simulink model "Final_Implementation"  (R2025b)
settings: Solver=ode4  StartTime=0.0  StopTime=10.0  FixedStep=2e-4  RelTol=1e-3  EnableMultiTasking=on
undefined symbols (not defined in the file or in its folder): P, Q_local, Q_opt_scaled, Q_OPT_scaled, T_S, x_0
libraries: simulink x4, dspsigops x3, SignalEditorBlockLib x1
settings Model: SimulationMode=rapid-accelerator  SILPILSystemUnderTest=refmodels  SILPILSimulationModeTopModel=rapid-accelerator  CodeVerificationMode=processor-in-the-loop (pil)  ExtModeTrigDuration=2  ExplicitPartitioning=on  Creator=nabil  LastModifiedBy=ouka1
settings SolverCC: AllowMultiTaskInputOutput=on  ConcurrentTasks=on  PositivePriorityOrder=on  AutoInsertRateTranBlk=on
settings OptimizationCC: StrengthReduction=on  PassReuseOutputArgsAs=Individual arguments  ZeroExternalMemoryAtStartup=off  ZeroInternalMemoryAtStartup=off  MaxStackSize=200000  OptimizeBlockOrder=speed  OptimizationPriority=Speed  OptimizationCustomize=off  MultiThreadedLoops=on  AutoScheduleForLoops=on  EfficientTunableParamExpr=on
settings DebuggingCC: ParameterTunabilityLossMsg=error
settings HardwareCC: ProdBitPerLong=64.0  ProdLargestAtomicInteger=LongLong  ProdLargestAtomicFloat=Double  ProdLongLongMode=on  ProdHWDeviceType=ARM Compatible->ARM Cortex-A (64-bit)
settings ModelReferenceCC: PropagateVarSize=During execution
settings SFSimCC: SimUserIncludeDirs=./Simulation_ert_rtw/
settings SFSimCC: SimUserSources=|
  | functions.c
  | Simulation.c
  | Simulation_data.c
settings RTWCC: SystemTargetFile=ert.tlc  HardwareBoard=Raspberry Pi (64bit)  TLCOptions="-aInlineSetEventsForThisBaseRateFcn=TLC_FALSE -aSuppressMultiTaskScheduler=TLC_FALSE  -aRateBasedStepFcn=0"  TemplateMakefile=ert_default_tmf  CustomInclude=./Simulation_ert_rtw/  Toolchain=GNU GCC Embedded Linux  BuildConfiguration=Faster Runs  IncludeHyperlinkInReport=on  GenerateCodeMetricsReport=on  Description=Embedded Coder
settings RTWCC: CustomHeaderCode=|
  | functions.h
  | Simulation.h
settings RTWCC: CustomSource=|
  | functions.c
  | Simulation.c
settings CodeAppCC: ForceParamTrailComments=on  IgnoreCustomStorageClasses=off  OperatorAnnotations=on  SimulinkDataObjDesc=on  SFDataObjDesc=on  InsertBlockDesc=on
settings ERTTargetCC: ExtModeTransport=2.0  ExtModeStaticAlloc=on  ExtModeMexFile=ext_xcp  ExtModeIntrfLevel=Level2 - Open  InlinedParameterPlacement=Hierarchical  CodeReplacementLibrary=ARM Cortex-A CMSIS  SupportNonFinite=off  SupportVariableSizeSignals=on  InstructionSetFMA=on  OptimizeReductions=on

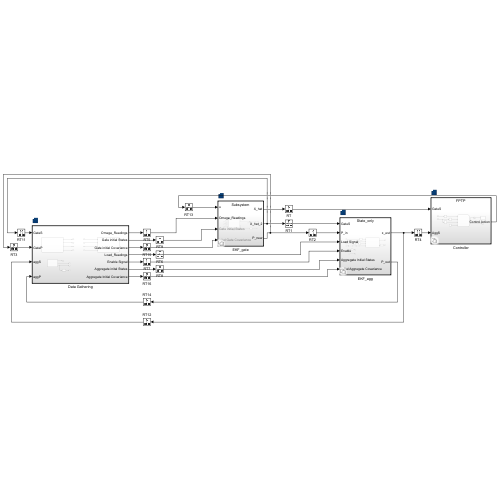
[thumbnail: Simulink's stored preview of the top-level diagram]
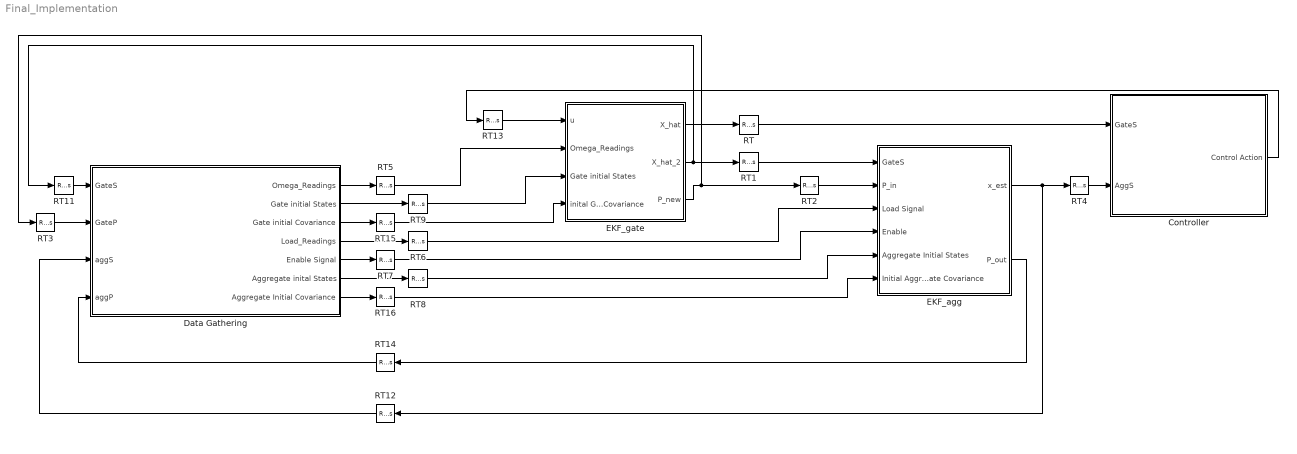
== system Final_Implementation ==
  Controller : Subsystem  TreatAsAtomicUnit=on  Variant=on  EmptyChoice=on
  Data Gathering : Subsystem  TreatAsAtomicUnit=on  SystemSampleTime=2e-3
  EKF_agg : Subsystem  TreatAsAtomicUnit=on  Variant=on  EmptyChoice=on
  EKF_gate : Subsystem  TreatAsAtomicUnit=on  Variant=on  EmptyChoice=on
  RT : RateTransition  Deterministic=off  OutPortSampleTime=0.005
  RT{1..2,6..8,16} (6 alike) : RateTransition  Deterministic=off  OutPortSampleTime=0.001
  RT{3,11..12,14} (4 alike) : RateTransition  Deterministic=off  OutPortSampleTime=0.002
  RT{5,9,13,15} (4 alike) : RateTransition  Deterministic=off  OutPortSampleTime=0.0002
  RT4 : RateTransition  Deterministic=off  OutPortSampleTime=0.005
  wires:
  Data Gathering/1(Omega_Readings) -> RT5/1
  Data Gathering/4(Load_Readings) -> RT6/1
  Data Gathering/5(Enable Signal) -> RT7/1
  Data Gathering/6(Aggregate inital States) -> RT8/1
  Data Gathering/2(Gate initial States) -> RT9/1
  RT11/1 -> Data Gathering/1(GateS)
  RT12/1 -> Data Gathering/3(aggS)
  RT3/1 -> Data Gathering/2(GateP)
  RT14/1 -> Data Gathering/4(aggP)
  Data Gathering/3(Gate initial Covariance) -> RT15/1
  Data Gathering/7(Aggregate Initial Covariance) -> RT16/1
  RT/1 -> Controller/1(GateS)
  RT4/1 -> Controller/2(AggS)
  Controller/1(Control Action) -> RT13/1
  RT1/1 -> EKF_agg/1(GateS)
  RT2/1 -> EKF_agg/2(P_in)
  RT6/1 -> EKF_agg/3(Load Signal)
  RT7/1 -> EKF_agg/4(Enable)
  RT8/1 -> EKF_agg/5(Aggregate Initial States)
  RT16/1 -> EKF_agg/6(Initial Aggregate Covariance)
  EKF_agg/1(x_est) -> RT4/1, RT12/1
  EKF_agg/2(P_out) -> RT14/1
  RT13/1 -> EKF_gate/1(u)
  RT5/1 -> EKF_gate/2(Omega_Readings)
  RT9/1 -> EKF_gate/3(Gate initial States)
  RT15/1 -> EKF_gate/4(inital Gate Covariance)
  EKF_gate/1(X_hat) -> RT/1
  EKF_gate/2(X_hat_2) -> RT1/1, RT11/1
  EKF_gate/3(P_new) -> RT2/1, RT3/1

== system Final_Implementation/Controller ==
  GateS : Inport
  AggS : Inport  Port=2
  FPTP : Subsystem  VariantControl=Controller==1
  MPC : Subsystem  TreatAsAtomicUnit=on  SystemSampleTime=0.005  VariantControl=Controller==0
  Control Action : Outport

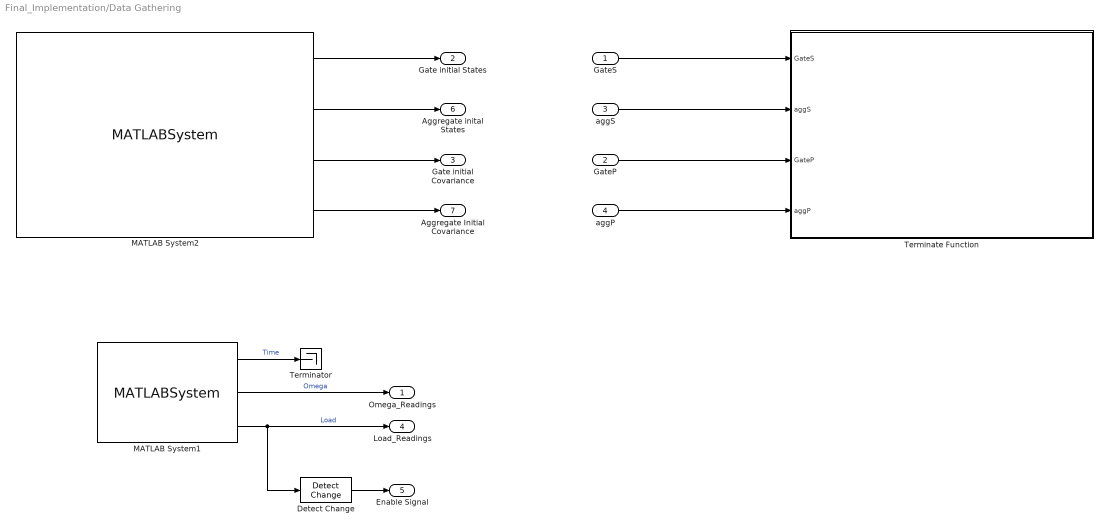
== system Final_Implementation/Data Gathering ==
  GateS : Inport
  GateP : Inport  Port=2
  aggS : Inport  Port=3
  aggP : Inport  Port=4
  Detect Change : simulink/Logic and Bit Operations/Detect Change  vinit=0  OutDataTypeStr=boolean
  MATLAB System1 : MATLABSystem  System=SerialReadBlock  SimulateUsing=Code generation
      mask Type: SerialReadBlock
  MATLAB System2 : MATLABSystem  System=LastStateInitializer  FileName=sim_data.csv  SimulateUsing=Code generation
      mask Type: LastStateInitializer
  Terminate Function : Subsystem  TreatAsAtomicUnit=on
  Terminator : Terminator
  Omega_Readings : Outport
  Gate initial States : Outport  Port=2
  Gate initial Covariance : Outport  Port=3
  Load_Readings : Outport  Port=4
  Enable Signal : Outport  Port=5
  Aggregate inital States : Outport  Port=6
  Aggregate Initial Covariance : Outport  Port=7
  wires:
  MATLAB System1/2 -> Omega_Readings/1  "Omega"
  MATLAB System1/3 -> Detect Change/1, Load_Readings/1  "Load"
  Detect Change/1 -> Enable Signal/1
  MATLAB System2/1 -> Gate initial States/1
  MATLAB System2/2 -> Aggregate inital States/1
  MATLAB System2/3 -> Gate initial Covariance/1
  MATLAB System2/4 -> Aggregate Initial Covariance/1
  aggS/1 -> Terminate Function/2(aggS)
  GateP/1 -> Terminate Function/3(GateP)
  GateS/1 -> Terminate Function/1(GateS)
  aggP/1 -> Terminate Function/4(aggP)
  MATLAB System1/1 -> Terminator/1  "Time"

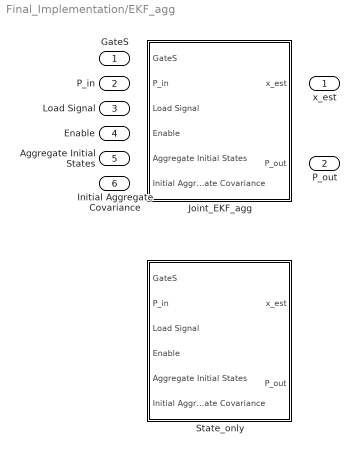
== system Final_Implementation/EKF_agg ==
  GateS : Inport
  P_in : Inport  Port=2
  Load Signal : Inport  Port=3
  Enable : Inport  Port=4
  Aggregate Initial States : Inport  Port=5
  Initial Aggregate Covariance : Inport  Port=6
  Joint_EKF_agg : Subsystem  TreatAsAtomicUnit=on  SystemSampleTime=1e-3  VariantControl=Estimator==0
  State_only : Subsystem  TreatAsAtomicUnit=on  VariantControl=Estimator==1
  x_est : Outport
  P_out : Outport  Port=2

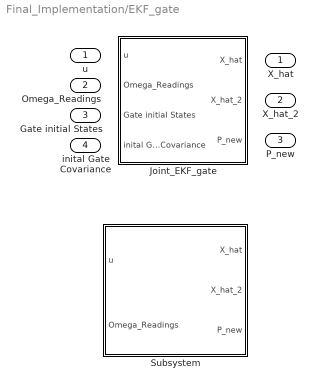
== system Final_Implementation/EKF_gate ==
  u : Inport
  Omega_Readings : Inport  Port=2
  Gate initial States : Inport  Port=3
  inital Gate Covariance : Inport  Port=4
  Joint_EKF_gate : Subsystem  TreatAsAtomicUnit=on  SystemSampleTime=2e-4  VariantControl=Estimator==0
  Subsystem : Subsystem  TreatAsAtomicUnit=on  VariantControl=Estimator==1
  X_hat : Outport
  X_hat_2 : Outport  Port=2
  P_new : Outport  Port=3

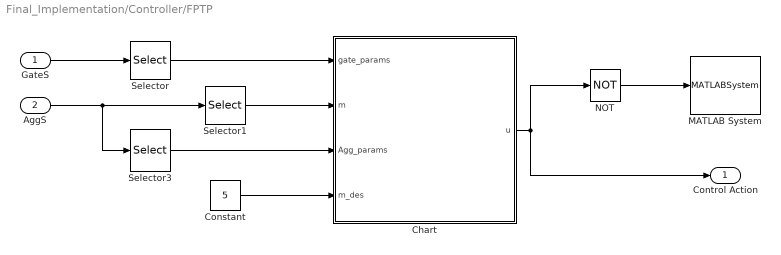
== system Final_Implementation/Controller/FPTP ==
  GateS : Inport
  AggS : Inport  Port=2
  Chart : Stateflow chart  TreatAsAtomicUnit=on
      settings: PortSchema="{\"entries\":[{\"content\":{\"sides\":[{\"content\":{\"connectorIds\":[\"In1\",\"In3\",\"In2\",\"In4\"]},\"type\":\"ConnectorPlacement.EquallySpacedRectSide\",\"uuid\":\"c09b967c-3e4e-4bac-bda4-fda1bd96a736\"},{\"content\":{\"connectorIds\":[\"Out1\"],\"side\":\"RIGHT\"},\"type\":\"ConnectorPlacement.EquallySpacedRectSide\",\"uuid\":\"db87db1d-7eac-4fd3-9563-2d6b00b990a6\"},{\"content\":{\"side\":\"TOP\"},\"type\":\"ConnectorPlacement.EquallySpacedRectSide\",\"uuid\":\"64da0432-1b95-42e2-a853-d892c1769434\"}]},\"type\":\"ConnectorPlacement.EquallySpacedConnector\",\"uuid\":\"e785f849-6cb9-45a7-bfa8-d41e67ce6963\"}],\"packageUris\":[\"http://schema.mathworks.com/mf0/Connector/R2020b\"],\"version\":\"1.0\"}"
  Constant : Constant  Value=5
  MATLAB System : MATLABSystem  System=GateDriver  SimulateUsing=Code generation
      mask Type: GateDriver
  NOT : Logic  Operator=NOT  IconShape=distinctive  AllPortsSameDT=off  OutDataTypeStr=boolean
  Selector : Selector  InputPortWidth=6  IndexOptions=Index vector (dialog)  Indices=[5 6]  OutputSizes=1
  Selector1 : Selector  InputPortWidth=9  IndexOptions=Index vector (dialog)  Indices=2  OutputSizes=1
  Selector3 : Selector  InputPortWidth=9  IndexOptions=Index vector (dialog)  Indices=[5:9]  OutputSizes=1
  Control Action : Outport
  wires:
  GateS/1 -> Selector/1
  Selector/1 -> Chart/1(gate_params)
  AggS/1 -> Selector3/1, Selector1/1
  Selector1/1 -> Chart/3(m)
  Constant/1 -> Chart/4(m_des)
  Selector3/1 -> Chart/2(Agg_params)
  NOT/1 -> MATLAB System/1
  Chart/1(u) -> NOT/1, Control Action/1

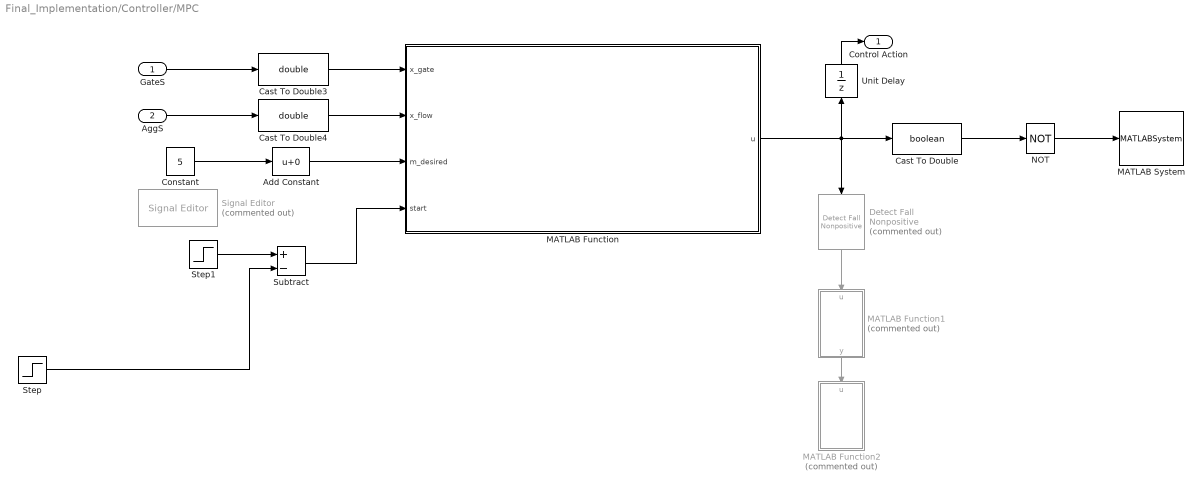
== system Final_Implementation/Controller/MPC ==
  GateS : Inport
  AggS : Inport  Port=2
  Add Constant : Bias  SaturateOnIntegerOverflow=off
  Cast To Double : DataTypeConversion  OutDataTypeStr=boolean  SaturateOnIntegerOverflow=off  RndMeth=Floor
  Cast To Double3 : DataTypeConversion  OutDataTypeStr=double  SaturateOnIntegerOverflow=off  RndMeth=Floor
  Cast To Double4 : DataTypeConversion  OutDataTypeStr=double  SaturateOnIntegerOverflow=off  RndMeth=Floor
  Constant : Constant  Value=5
  Detect Fall Nonpositive : simulink/Logic and Bit Operations/Detect Fall Nonpositive  Commented=on  vinit=0  OutDataTypeStr=boolean
  MATLAB Function : MATLAB Function  TreatAsAtomicUnit=on
  MATLAB Function1 : MATLAB Function  Commented=on  TreatAsAtomicUnit=on
  MATLAB Function2 : MATLAB Function  Commented=on  TreatAsAtomicUnit=on
  MATLAB System : MATLABSystem  System=GateDriver  SimulateUsing=Code generation
      mask Type: GateDriver
  NOT : Logic  Operator=NOT  IconShape=distinctive  AllPortsSameDT=off  OutDataTypeStr=boolean
  Signal Editor : SignalEditorBlockLib/Signal Editor  Commented=on  FileName=untitled.mat  ActiveScenario=Scenario  ActiveSignal=Signal 1  IsBus=off  OutputBusObjectStr=Bus: BusObject  SampleTime=0.005  ZeroCross=off  OutputAfterFinalValue=Setting to zero  Unit=inherit  PreserveSignalName=on  ApplySigPropsToAllScenarios=on  ApplySigPropsToAllSignals=off  SignalPropertySource=Dialog parameters
  Step : Step  Time=5e-3  Before=1  After=0
  Step1 : Step  Time=15e-3  Before=1  After=0
  Subtract : Sum  Inputs=+-
  Unit Delay : UnitDelay  SampleTime=0.005  HasFrameUpgradeWarning=on
  Control Action : Outport
  wires:
  Cast To Double4/1 -> MATLAB Function/2(x_flow)
  Constant/1 -> Add Constant/1
  Cast To Double3/1 -> MATLAB Function/1(x_gate)
  Unit Delay/1 -> Control Action/1
  AggS/1 -> Cast To Double4/1
  GateS/1 -> Cast To Double3/1
  Cast To Double/1 -> NOT/1
  NOT/1 -> MATLAB System/1
  MATLAB Function/1(u) -> Detect Fall Nonpositive/1, Cast To Double/1, Unit Delay/1
  Detect Fall Nonpositive/1 -> MATLAB Function1/1(u)
  MATLAB Function1/1(y) -> MATLAB Function2/1(u)
  Step1/1 -> Subtract/1
  Step/1 -> Subtract/2
  Subtract/1 -> MATLAB Function/4(start)
  Add Constant/1 -> MATLAB Function/3(m_desired)

== system Final_Implementation/Data Gathering/Terminate Function ==
  GateS : Inport
  aggS : Inport  Port=2
  GateP : Inport  Port=3
  aggP : Inport  Port=4
  Event Listener : EventListener  DisableCoverage=on  EventType=Terminate  EventName=reset
  MATLAB System : MATLABSystem  System=LoggerBlock  SimulateUsing=Code generation
      mask Type: LoggerBlock
  wires:
  GateP/1 -> MATLAB System/3
  aggP/1 -> MATLAB System/4
  GateS/1 -> MATLAB System/1
  aggS/1 -> MATLAB System/2

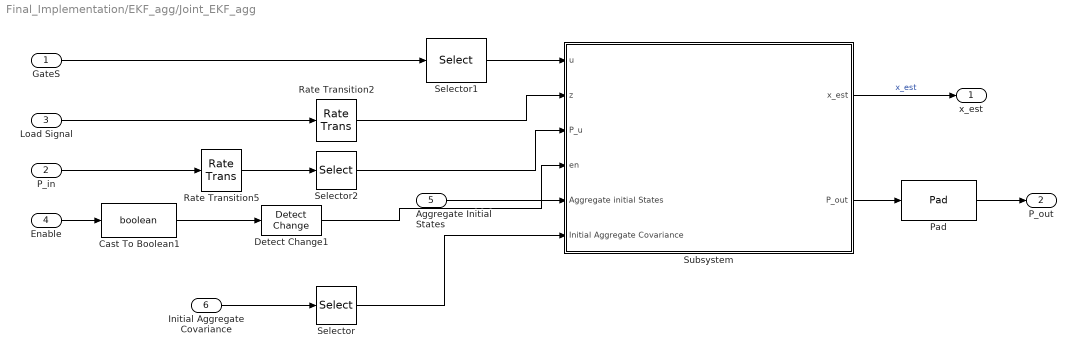
== system Final_Implementation/EKF_agg/Joint_EKF_agg ==
  GateS : Inport
  P_in : Inport  Port=2
  Load Signal : Inport  Port=3
  Enable : Inport  Port=4
  Aggregate Initial States : Inport  Port=5
  Initial Aggregate Covariance : Inport  Port=6
  Cast To Boolean1 : DataTypeConversion  OutDataTypeStr=boolean  SaturateOnIntegerOverflow=off  RndMeth=Floor
  Detect Change1 : simulink/Logic and Bit Operations/Detect Change  vinit=0  OutDataTypeStr=boolean
  Pad : dspsigops/Pad  padAlong=Columns and rows  dimsToPad=1  valSrc=Specify via dialog  padVal=0  spec=Output size  padNumOutRowsSpecMethod=User-specified  numOutRows=9  padNumOutColsSpecMethod=User-specified  numOutCols=9  isVarDimsMode=off  padBeginning=0  padEnd=0  outSizeMode=User-specified  outSize=1  padSigAt=End  trunc_flag=None  roundingMode=Floor  overflowMode=off  truncOrWrapMode=Truncate  wrap_flag=None
  Rate Transition2 : RateTransition
  Rate Transition5 : RateTransition
  Selector : Selector  NumberOfDimensions=2  InputPortWidth=3  IndexOptions=Index vector (dialog),Index vector (dialog)  Indices=[1:7],[1:7]  OutputSizes=1,1
  Selector1 : Selector  InputPortWidth=6  IndexOptions=Index vector (dialog)  Indices=1  OutputSizes=1
  Selector2 : Selector  NumberOfDimensions=2  InputPortWidth=7,7  IndexOptions=Index vector (dialog),Index vector (dialog)  Indices=1,1  OutputSizes=1,1
  Subsystem : Subsystem
  x_est : Outport
  P_out : Outport  Port=2
  wires:
  Subsystem/1(x_est) -> x_est/1  "x_est"
  Subsystem/2(P_out) -> Pad/1
  Enable/1 -> Cast To Boolean1/1
  Rate Transition2/1 -> Subsystem/2(z)
  Cast To Boolean1/1 -> Detect Change1/1
  P_in/1 -> Rate Transition5/1
  Rate Transition5/1 -> Selector2/1
  Selector1/1 -> Subsystem/1(u)
  Load Signal/1 -> Rate Transition2/1
  Detect Change1/1 -> Subsystem/4(en)
  Selector2/1 -> Subsystem/3(P_u)
  Aggregate Initial States/1 -> Subsystem/5(Aggregate initial States)
  GateS/1 -> Selector1/1
  Initial Aggregate Covariance/1 -> Selector/1
  Selector/1 -> Subsystem/6(Initial Aggregate Covariance)
  Pad/1 -> P_out/1

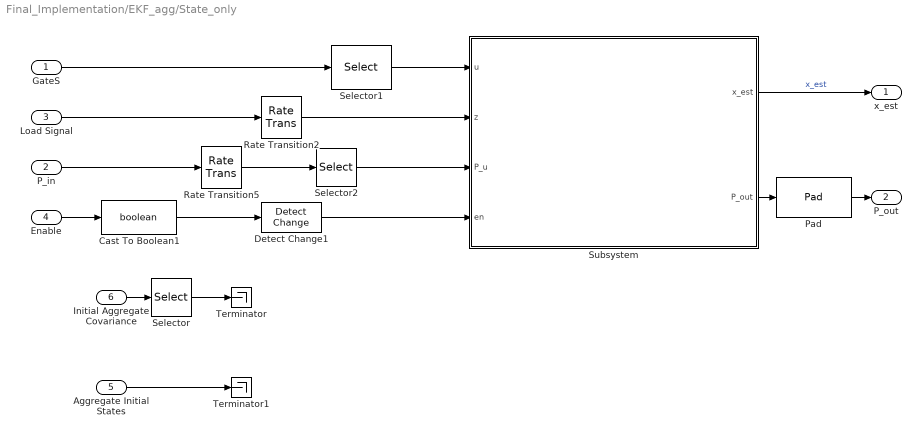
== system Final_Implementation/EKF_agg/State_only ==
  GateS : Inport
  P_in : Inport  Port=2
  Load Signal : Inport  Port=3
  Enable : Inport  Port=4
  Aggregate Initial States : Inport  Port=5
  Initial Aggregate Covariance : Inport  Port=6
  Cast To Boolean1 : DataTypeConversion  OutDataTypeStr=boolean  SaturateOnIntegerOverflow=off  RndMeth=Floor
  Detect Change1 : simulink/Logic and Bit Operations/Detect Change  vinit=0  OutDataTypeStr=boolean
  Pad : dspsigops/Pad  padAlong=Columns and rows  dimsToPad=1  valSrc=Specify via dialog  padVal=0  spec=Output size  padNumOutRowsSpecMethod=User-specified  numOutRows=9  padNumOutColsSpecMethod=User-specified  numOutCols=9  isVarDimsMode=off  padBeginning=0  padEnd=0  outSizeMode=User-specified  outSize=1  padSigAt=End  trunc_flag=None  roundingMode=Floor  overflowMode=off  truncOrWrapMode=Truncate  wrap_flag=None
  Rate Transition2 : RateTransition
  Rate Transition5 : RateTransition
  Selector : Selector  NumberOfDimensions=2  InputPortWidth=3  IndexOptions=Index vector (dialog),Index vector (dialog)  Indices=[1:4],[1:4]  OutputSizes=1,1
  Selector1 : Selector  InputPortWidth=6  IndexOptions=Index vector (dialog)  Indices=1  OutputSizes=1
  Selector2 : Selector  NumberOfDimensions=2  InputPortWidth=7,7  IndexOptions=Index vector (dialog),Index vector (dialog)  Indices=1,1  OutputSizes=1,1
  Subsystem : Subsystem
  Terminator : Terminator
  Terminator1 : Terminator
  x_est : Outport
  P_out : Outport  Port=2
  wires:
  GateS/1 -> Selector1/1
  Rate Transition2/1 -> Subsystem/2(z)
  Detect Change1/1 -> Subsystem/4(en)
  Pad/1 -> P_out/1
  Subsystem/2(P_out) -> Pad/1
  Cast To Boolean1/1 -> Detect Change1/1
  Initial Aggregate Covariance/1 -> Selector/1
  Load Signal/1 -> Rate Transition2/1
  Rate Transition5/1 -> Selector2/1
  Selector/1 -> Terminator/1
  Selector1/1 -> Subsystem/1(u)
  Subsystem/1(x_est) -> x_est/1  "x_est"
  Selector2/1 -> Subsystem/3(P_u)
  Aggregate Initial States/1 -> Terminator1/1
  P_in/1 -> Rate Transition5/1
  Enable/1 -> Cast To Boolean1/1

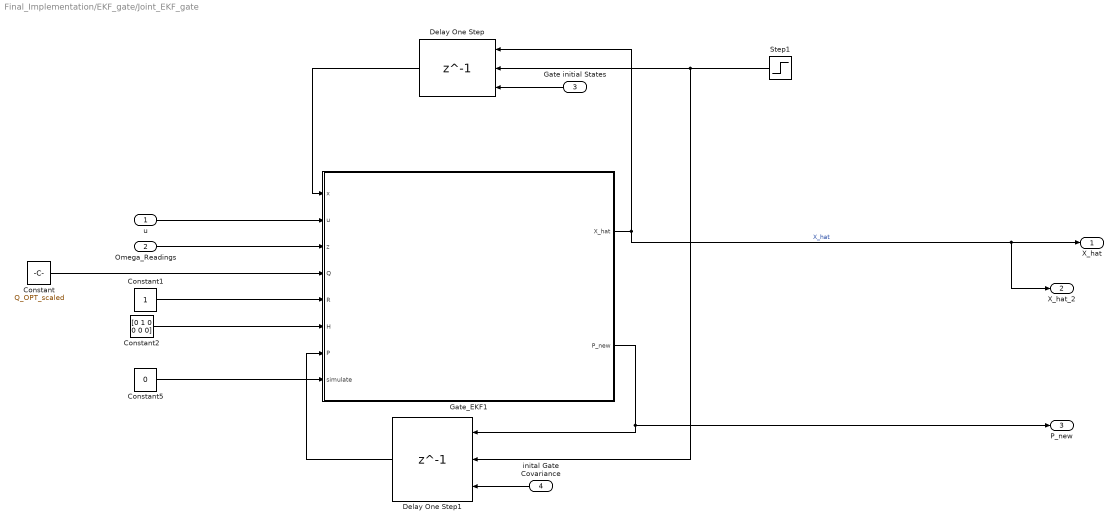
== system Final_Implementation/EKF_gate/Joint_EKF_gate ==
  u : Inport
  Omega_Readings : Inport  Port=2
  Gate initial States : Inport  Port=3
  inital Gate Covariance : Inport  Port=4
  Constant : Constant  Value=Q_OPT_scaled
  Constant1 : Constant
  Constant2 : Constant  Value=[0 1 0 0 0 0]
  Constant5 : Constant  Value=0
  Delay One Step : Delay  DelayLength=1  InitialConditionSource=Input port  ExternalReset=Falling
      settings: InputPortMap=u0,r5,p4
  Delay One Step1 : Delay  DelayLength=1  InitialConditionSource=Input port  InitialCondition=diag([1e-6 1e-6 0.1 0.1 0.1 1e-6 1e-6])  ExternalReset=Falling
      settings: InputPortMap=u0,r5,p4
  Gate_EKF1 : MATLAB Function  TreatAsAtomicUnit=on
  Step1 : Step  Time=2.1e-3  Before=1  After=0
  X_hat : Outport
  X_hat_2 : Outport  Port=2
  P_new : Outport  Port=3
  wires:
  Constant1/1 -> Gate_EKF1/5(R)
  Constant5/1 -> Gate_EKF1/8(simulate)
  Gate_EKF1/1(X_hat) -> X_hat_2/1, X_hat/1, Delay One Step/1  "X_hat"
  Delay One Step1/1 -> Gate_EKF1/7(P)
  Gate_EKF1/2(P_new) -> P_new/1, Delay One Step1/1
  u/1 -> Gate_EKF1/2(u)
  Constant2/1 -> Gate_EKF1/6(H)
  Constant/1 -> Gate_EKF1/4(Q)
  Omega_Readings/1 -> Gate_EKF1/3(z)
  Delay One Step/1 -> Gate_EKF1/1(x)
  Gate initial States/1 -> Delay One Step/3
  Step1/1 -> Delay One Step1/2, Delay One Step/2
  inital Gate Covariance/1 -> Delay One Step1/3

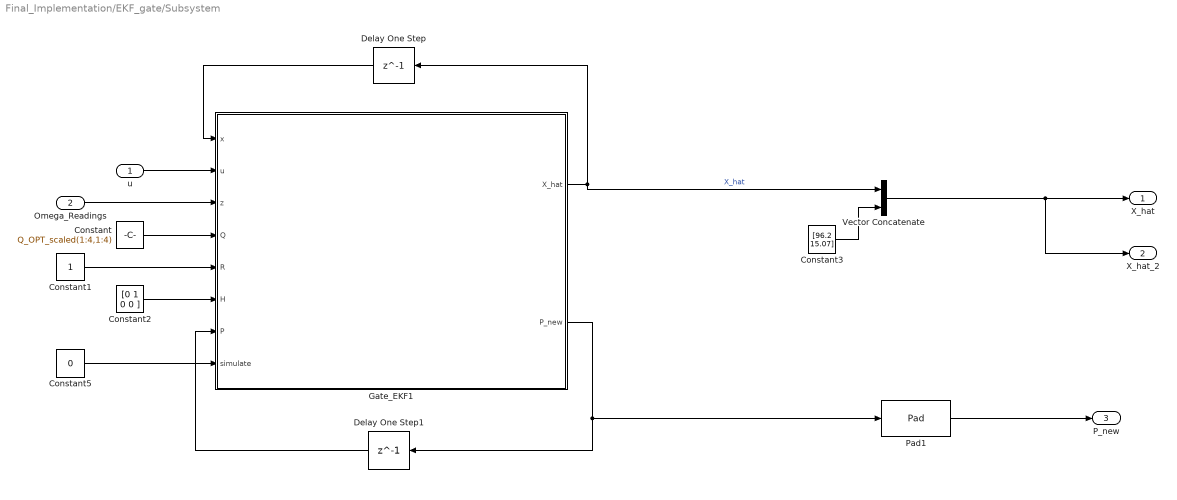
== system Final_Implementation/EKF_gate/Subsystem ==
  u : Inport
  Omega_Readings : Inport  Port=2
  Constant : Constant  Value=Q_OPT_scaled(1:4,1:4)
  Constant1 : Constant
  Constant2 : Constant  Value=[0 1 0 0 ]
  Constant3 : Constant  Value=[96.2 15.07]
  Constant5 : Constant  Value=0
  Delay One Step : Delay  DelayLength=1  InitialCondition=[0 0 9*1.01325e5 1.01325e5]'
  Delay One Step1 : Delay  DelayLength=1  InitialCondition=diag([1e-6 1e-6 0.1 0.1] )
  Gate_EKF1 : MATLAB Function  TreatAsAtomicUnit=on
  Pad1 : dspsigops/Pad  padAlong=Columns and rows  dimsToPad=1  valSrc=Specify via dialog  padVal=0  spec=Output size  padNumOutRowsSpecMethod=User-specified  numOutRows=6  padNumOutColsSpecMethod=User-specified  numOutCols=6  isVarDimsMode=off  padBeginning=0  padEnd=0  outSizeMode=User-specified  outSize=1  padSigAt=End  trunc_flag=None  roundingMode=Floor  overflowMode=off  truncOrWrapMode=Truncate  wrap_flag=None
  Vector Concatenate : Concatenate
  X_hat : Outport
  X_hat_2 : Outport  Port=2
  P_new : Outport  Port=3
  wires:
  Omega_Readings/1 -> Gate_EKF1/3(z)
  Delay One Step1/1 -> Gate_EKF1/7(P)
  Constant2/1 -> Gate_EKF1/6(H)
  u/1 -> Gate_EKF1/2(u)
  Gate_EKF1/1(X_hat) -> Vector Concatenate/1, Delay One Step/1  "X_hat"
  Constant1/1 -> Gate_EKF1/5(R)
  Constant/1 -> Gate_EKF1/4(Q)
  Gate_EKF1/2(P_new) -> Pad1/1, Delay One Step1/1
  Delay One Step/1 -> Gate_EKF1/1(x)
  Constant5/1 -> Gate_EKF1/8(simulate)
  Vector Concatenate/1 -> X_hat_2/1, X_hat/1
  Pad1/1 -> P_new/1
  Constant3/1 -> Vector Concatenate/2

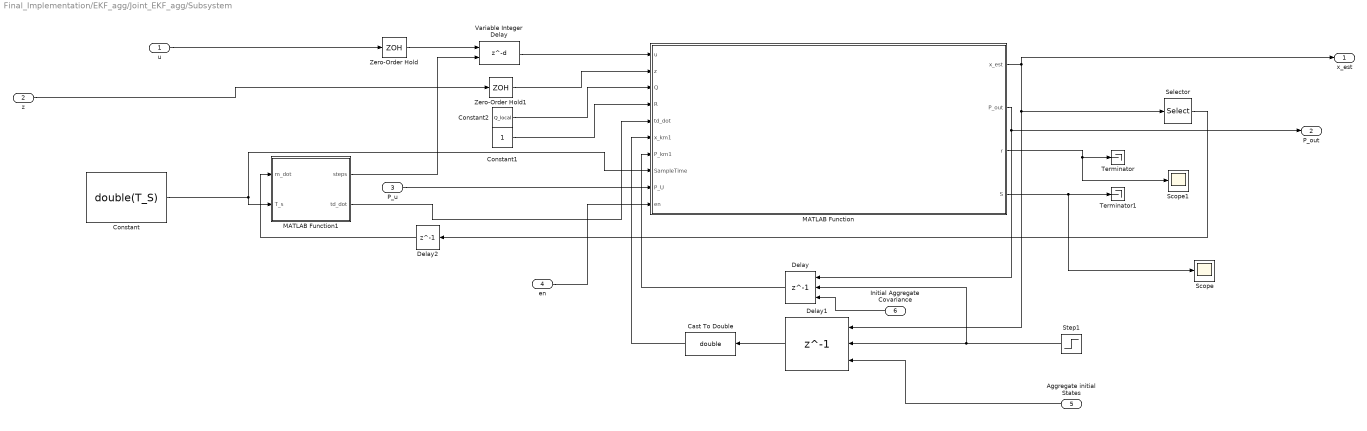
== system Final_Implementation/EKF_agg/Joint_EKF_agg/Subsystem ==
  u : Inport
  z : Inport  Port=2
  P_u : Inport  Port=3
  en : Inport  Port=4
  Aggregate initial States : Inport  Port=5
  Initial Aggregate Covariance : Inport  Port=6
  Cast To Double : DataTypeConversion  OutDataTypeStr=double  SaturateOnIntegerOverflow=off  RndMeth=Floor
  Constant : Constant  Value=double(T_S)  OutDataTypeStr=double
  Constant1 : Constant
  Constant2 : Constant  Value=Q_local
  Delay : Delay  DelayLength=1  InitialConditionSource=Input port  InitialCondition=P  ExternalReset=Falling  SampleTime=T_S
      settings: InputPortMap=u0,r5,p4
  Delay1 : Delay  DelayLength=1  InitialConditionSource=Input port  InitialCondition=x_0  ExternalReset=Falling  SampleTime=T_S
      settings: InputPortMap=u0,r5,p4
  Delay2 : Delay  DelayLength=1  InputProcessing=Columns as channels (frame based)
  MATLAB Function : MATLAB Function  TreatAsAtomicUnit=on
  MATLAB Function1 : MATLAB Function  TreatAsAtomicUnit=on
  Scope : Scope
  Scope1 : Scope
  Selector : Selector  InputPortWidth=9  IndexOptions=Index vector (dialog)  Indices=1  OutputSizes=1
  Step1 : Step  Time=2.1e-3  Before=1  After=0
  Terminator : Terminator
  Terminator1 : Terminator
  Variable Integer Delay : Delay  DelayLengthSource=Input port  DelayLengthUpperLimit=500
      settings: InputPortMap=u0,p1
  Zero-Order Hold : ZeroOrderHold  SampleTime=T_S
  Zero-Order Hold1 : ZeroOrderHold  SampleTime=T_S
  x_est : Outport  OutDataTypeStr=double
  P_out : Outport  Port=2
  wires:
  Constant2/1 -> MATLAB Function/3(Q)
  en/1 -> MATLAB Function/10(en)
  Delay1/1 -> Cast To Double/1
  MATLAB Function1/2(td_dot) -> MATLAB Function/5(td_dot)
  Delay2/1 -> MATLAB Function1/1(m_dot)
  Selector/1 -> Delay2/1
  Zero-Order Hold1/1 -> MATLAB Function/2(z)
  MATLAB Function/1(x_est) -> x_est/1, Selector/1, Delay1/1
  z/1 -> Zero-Order Hold1/1
  Variable Integer Delay/1 -> MATLAB Function/1(u)
  MATLAB Function/3(r) -> Terminator/1, Scope1/1
  u/1 -> Zero-Order Hold/1
  MATLAB Function/4(S) -> Terminator1/1, Scope/1
  MATLAB Function1/1(steps) -> Variable Integer Delay/2
  Zero-Order Hold/1 -> Variable Integer Delay/1
  P_u/1 -> MATLAB Function/9(P_U)
  Cast To Double/1 -> MATLAB Function/6(x_km1)
  Constant1/1 -> MATLAB Function/4(R)
  MATLAB Function/2(P_out) -> P_out/1, Delay/1
  Delay/1 -> MATLAB Function/7(P_km1)
  Constant/1 -> MATLAB Function/8(SampleTime), MATLAB Function1/2(T_s)
  Aggregate initial States/1 -> Delay1/3
  Step1/1 -> Delay/2, Delay1/2
  Initial Aggregate Covariance/1 -> Delay/3

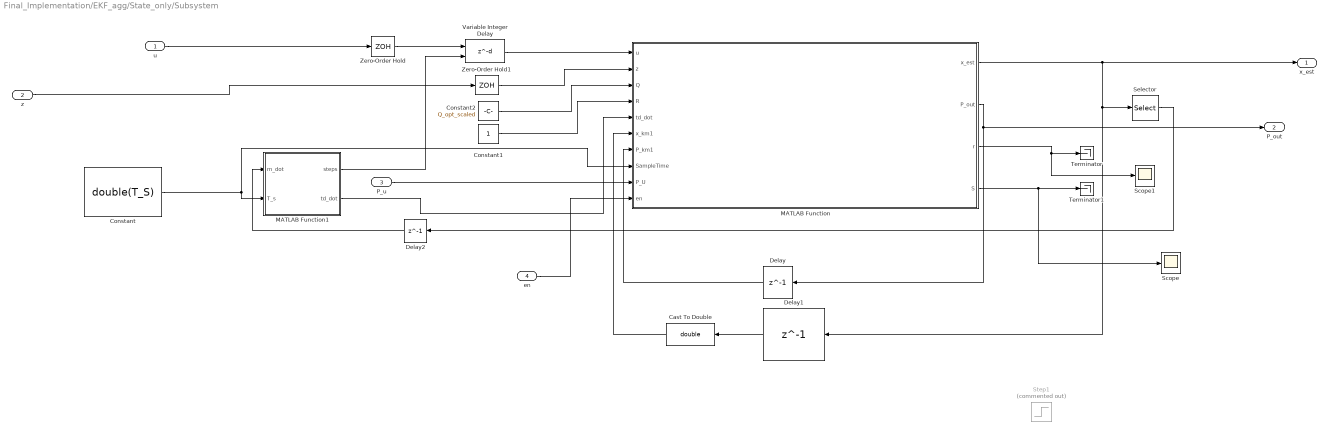
== system Final_Implementation/EKF_agg/State_only/Subsystem ==
  u : Inport
  z : Inport  Port=2
  P_u : Inport  Port=3
  en : Inport  Port=4
  Cast To Double : DataTypeConversion  OutDataTypeStr=double  SaturateOnIntegerOverflow=off  RndMeth=Floor
  Constant : Constant  Value=double(T_S)  OutDataTypeStr=double
  Constant1 : Constant
  Constant2 : Constant  Value=Q_opt_scaled
  Delay : Delay  DelayLength=1  InitialCondition=zeros(4)  SampleTime=T_S
  Delay1 : Delay  DelayLength=1  InitialCondition=x_0  SampleTime=T_S
  Delay2 : Delay  DelayLength=1  InputProcessing=Columns as channels (frame based)
  MATLAB Function : MATLAB Function  TreatAsAtomicUnit=on
  MATLAB Function1 : MATLAB Function  TreatAsAtomicUnit=on
  Scope : Scope
  Scope1 : Scope
  Selector : Selector  InputPortWidth=9  IndexOptions=Index vector (dialog)  Indices=1  OutputSizes=1
  Step1 : Step  Commented=on  Time=2.1e-3  Before=1  After=0
  Terminator : Terminator
  Terminator1 : Terminator
  Variable Integer Delay : Delay  DelayLengthSource=Input port  DelayLengthUpperLimit=500
      settings: InputPortMap=u0,p1
  Zero-Order Hold : ZeroOrderHold  SampleTime=T_S
  Zero-Order Hold1 : ZeroOrderHold  SampleTime=T_S
  x_est : Outport  OutDataTypeStr=double
  P_out : Outport  Port=2
  wires:
  Constant2/1 -> MATLAB Function/3(Q)
  en/1 -> MATLAB Function/10(en)
  Delay1/1 -> Cast To Double/1
  MATLAB Function1/2(td_dot) -> MATLAB Function/5(td_dot)
  Delay2/1 -> MATLAB Function1/1(m_dot)
  Selector/1 -> Delay2/1
  Zero-Order Hold1/1 -> MATLAB Function/2(z)
  z/1 -> Zero-Order Hold1/1
  Variable Integer Delay/1 -> MATLAB Function/1(u)
  MATLAB Function/3(r) -> Terminator/1, Scope1/1
  u/1 -> Zero-Order Hold/1
  MATLAB Function/4(S) -> Terminator1/1, Scope/1
  MATLAB Function1/1(steps) -> Variable Integer Delay/2
  Zero-Order Hold/1 -> Variable Integer Delay/1
  P_u/1 -> MATLAB Function/9(P_U)
  Cast To Double/1 -> MATLAB Function/6(x_km1)
  Constant1/1 -> MATLAB Function/4(R)
  MATLAB Function/2(P_out) -> P_out/1, Delay/1
  Constant/1 -> MATLAB Function/8(SampleTime), MATLAB Function1/2(T_s)
  Delay/1 -> MATLAB Function/7(P_km1)
  MATLAB Function/1(x_est) -> x_est/1, Delay1/1, Selector/1

== matlab function Final_Implementation/EKF_agg/Joint_EKF_agg/Subsystem/MATLAB Function1 ==
  settings: updateMethod=DISCRETE  sampleTime=T_S
  data: m_dot input double; steps output int16; T_s input double; td_dot output double
function [steps, td_dot] = delay_steps(m_dot,T_s)
if m_dot>1e-3
    tk=0.162;
else
    tk=0.401;
end
[td, td_dot] = Transport_time(tk,T_s);
steps=int16(td/T_s);
end

== matlab function Final_Implementation/EKF_agg/State_only/Subsystem/MATLAB Function1 ==
  settings: updateMethod=DISCRETE  sampleTime=T_S
  data: m_dot input double; steps output int16; T_s input double; td_dot output double
function [steps, td_dot] = delay_steps(m_dot,T_s)
if m_dot>1e-3
    tk=0.162;
else
    tk=0.401;
end
[td, td_dot] = Transport_time(tk,T_s);
steps=int16(td/T_s);
end

== matlab function Final_Implementation/EKF_gate/Subsystem/Gate_EKF1 ==
  settings: updateMethod=DISCRETE  sampleTime=2e-4
  data: x input; u input; X_hat output; P_new output size=[4 4]; z input; Q input; R input; H input; P input; simulate input
function [X_hat,P_new] = EKF(x,u,z,Q,R,H,P,simulate)
%% prediction
    x_prior=x;
    for i=1:10
    x_prior = f_dynamics_Wo_DT(x_prior,u,2e-5);
    end
    J = Jacobian_Wo_DT(x,u,2e-4);
    if(simulate)
        X_hat = x_prior;
        P_new = zeros(4,4);
        return
    end
    P_prior = J * P * J' + Q;

%% innovation
    r = (z - H' * x_prior);
    S = (H'*P_prior*H+R);
    K = P_prior * H / S;
%% update
    I=eye(4);
    I_KH=I-K*H';
    P_new = I_KH*P*I_KH'+K*R*K';
    X_hat = x_prior + K * r;
end

== stateflow chart Final_Implementation/Controller/FPTP/Chart ==
  state Initialization
    during:
    delm=FPTPdelm(gate_params',Agg_params');
    u=1;
  state Open
    during:
    u=1;
  state Close
    during:
    u=0
  (default) -> Initialization
  Initialization -> Initialization [order 1] : [isnan(delm)]
  Open -> Close : [m_des-m<delm]
  Initialization -> Open [order 2] : after(3,tick)
  data: gate_params function_input; agg_params function_input; delM function_output; gate_params input; Agg_params input; m input; m_des input; u output =1; delm local
  function delM  = FPTPdelm(gate_params,agg_params):
    | function delM  = FPTPdelm(gate_params,agg_params)
    | %   Detailed explanation goes here
    | C_1=agg_params(1);
    | q=(C_1/0.03)*0.09*sin(0.8179-0.1701)*0.03^(1.5);
    | x_flow=[q 0 0 0 agg_params];
    | x_gate=[0.8179 0 9*1.013125e5 1.013125e5 9*1.013125e5 gate_params];
    | fprintf('x_flow = [');
    | delM=sim_batch(10,0,x_gate,x_flow)
    | 
    | %% logging data for debugging
    | for i = 1:length(x_flow)
    |     fprintf(' %f', x_flow(i));
    | end
    | fprintf(' ]\n');
    | fprintf('x_gate = [');
    | for i = 1:length(x_gate)
    |     fprintf(' %f', x_gate(i));
    | end
    | fprintf(' ]\n');
    | fprintf("%f\n",delM)
    | end

== matlab function Final_Implementation/Controller/MPC/MATLAB Function1 ==
  data: u input; y output
function y = fcn(u)
persistent fired count
if (isempty(fired))
    fired=0;
    count=0;
end
if u&&~fired
    fired =1;
end
if fired
    count=count+1;
end
if count>=1000
    y=1;
else
    y=0;
end

== matlab function Final_Implementation/Controller/MPC/MATLAB Function ==
  data: x_gate input; u output; x_flow input; m_desired input; start input
function u  = MPC(x_gate,x_flow,m_desired,start)
x_gate=[x_gate(1:2)' 9*(1.01325e5) x_gate(3:6)'];
% u=0;
[u] = NMPC(x_gate,x_flow,m_desired,start);

== matlab function Final_Implementation/Controller/MPC/MATLAB Function2 ==
  data: u input
function fcn(u)
if u
coder.ceval('raise', int32(15));
end

== matlab function Final_Implementation/EKF_gate/Joint_EKF_gate/Gate_EKF1 ==
  settings: updateMethod=DISCRETE  sampleTime=2e-4
  data: x input; u input; X_hat output; P_new output size=[6 6]; z input; Q input; R input; H input; P input; simulate input
function [X_hat,P_new] = EKF(x,u,z,Q,R,H,P,simulate)
persistent first_run 
if isempty(first_run)
    first_run = 1;
    P(5,5) = 1e-8;
    P(6,6) = 1e-8;

end
%% prediction
    x_prior=x;
    for i=1:10
    x_prior = f_dynamics(x_prior,u,2e-5);
    end
    J = Jacobian(x,u,2e-4);
    if(simulate)
        X_hat = x_prior;
        P_new = zeros(6,6);
        return
    end
    P_prior = J * P * J' + Q;

%% innovation
    r = (z - H' * x_prior);
    S = (H'*P_prior*H+R);
    K = P_prior * H / S;
%% update
    %I=eye(7);
    %I_KH=I-K*H';
    P_new = P_prior - K * H' * P_prior;
    X_hat = x_prior + K * r;
end

== matlab function Final_Implementation/EKF_agg/State_only/Subsystem/MATLAB Function ==
  settings: updateMethod=DISCRETE  sampleTime=T_S
  data: u input; x_est output double; z input; Q input; R input; td_dot input; x_km1 input; P_km1 input; SampleTime input; P_out output; r output; S output; P_U input; en input
function [x_est,P_out,r,S] = EKF(u,z,Q,R,td_dot,x_km1,P_km1,SampleTime,P_U,en)
[x_est,P_out,r,S] = NO_DT_EKF_delay_compensated(u,z,Q,R,td_dot,x_km1,P_km1,SampleTime,P_U,en);
end

== matlab function Final_Implementation/EKF_agg/Joint_EKF_agg/Subsystem/MATLAB Function ==
  settings: updateMethod=DISCRETE  sampleTime=T_S
  data: u input; x_est output double; z input; Q input; R input; td_dot input; x_km1 input; P_km1 input; SampleTime input; P_out output; r output; S output; P_U input; en input
function [x_est,P_out,r,S] = EKF(u,z,Q,R,td_dot,x_km1,P_km1,SampleTime,P_U,en)
[x_est,P_out,r,S] = EKF_delay_compensated(u,z,Q,R,td_dot,x_km1,P_km1,SampleTime,P_U,en);
end
